simulink model "ASMC_withoutBP"  (R2020b)
settings: Solver=ode45  StartTime=0.0  StopTime=20  FixedStep=0.001  RelTol=1e-3
settings Model: Creator=cyx  LastModifiedBy=cyx
settings SolverCC: AlgebraicLoopSolver=LineSearch
settings DataIOCC: ReturnWorkspaceOutputs=off

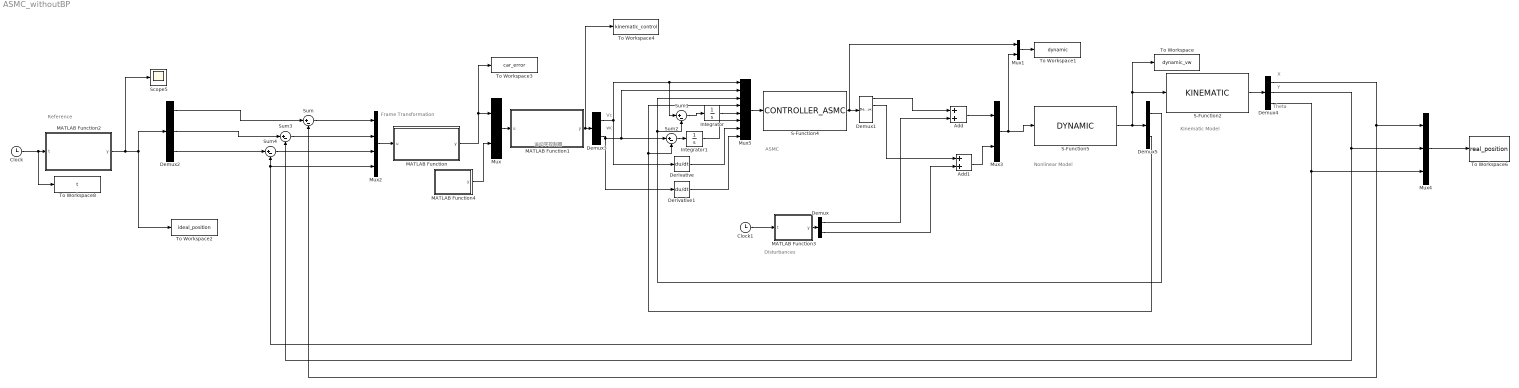
== system ASMC_withoutBP ==
  note: Y
  note: X
  note: Disturbances
  note: Reference
  note: Nonlinear Model
  note: ASMC
  note: 运动学控制器
  note: Kinematic Model
  note: Theta
  note: Vc
  note: Frame Transformation
  note: wc
  Add : Sum
  Add1 : Sum
  Clock : Clock
  Clock1 : Clock
  Demux : Demux  Outputs=2
  Demux1 : Demux
  Demux2 : Demux  Outputs=3
  Demux3 : Demux  Outputs=2
  Demux4 : Demux  Outputs=3
  Demux5 : Demux  Outputs=2
  Derivative : Derivative
  Derivative1 : Derivative
  Integrator : Integrator
  Integrator1 : Integrator
  MATLAB Function : MATLAB Function  TreatAsAtomicUnit=on
  MATLAB Function1 : MATLAB Function  TreatAsAtomicUnit=on
  MATLAB Function2 : MATLAB Function  TreatAsAtomicUnit=on
  MATLAB Function3 : MATLAB Function  TreatAsAtomicUnit=on
  MATLAB Function4 : MATLAB Function  TreatAsAtomicUnit=on
  Mux : Mux  Inputs=2
  Mux1 : Mux  Inputs=2
  Mux2 : Mux
  Mux3 : Mux  Inputs=2
  Mux4 : Mux  Inputs=3
  Mux5 : Mux  Inputs=8
  S-Function2 : S-Function  FunctionName=KINEMATIC  SFunctionDeploymentMode=off  EnableBusSupport=off
  S-Function4 : S-Function  FunctionName=CONTROLLER_ASMC  SFunctionDeploymentMode=off  EnableBusSupport=off
  S-Function5 : S-Function  FunctionName=DYNAMIC  SFunctionDeploymentMode=off  EnableBusSupport=off
  Scope5 : Scope
  Sum{,1..4} (5 alike) : Sum  Inputs=|+-
  To Workspace : ToWorkspace  VariableName=dynamic_vw  SampleTime=-1
  To Workspace1 : ToWorkspace  VariableName=dynamic  SampleTime=-1
  To Workspace2 : ToWorkspace  VariableName=ideal_position  SampleTime=-1
  To Workspace3 : ToWorkspace  VariableName=car_error  SampleTime=-1
  To Workspace4 : ToWorkspace  VariableName=kinematic_control  SampleTime=-1
  To Workspace6 : ToWorkspace  VariableName=real_position  SampleTime=-1
      settings: Save2DSignal=2-D array (concatenate along first dimension)
  To Workspace8 : ToWorkspace  VariableName=t  SampleTime=-1
  wires:
  Sum1/1 -> Integrator/1
  Demux3/1 -> Derivative/1, Sum1/1, Mux5/1
  Integrator1/1 -> Mux5/6
  Demux/2 -> Add1/2
  Integrator/1 -> Mux5/5
  Clock1/1 -> MATLAB Function3/1(t)
  Mux5/1 -> S-Function4/1
  Derivative1/1 -> Mux5/8
  Derivative/1 -> Mux5/7
  Sum2/1 -> Integrator1/1
  Demux3/2 -> Derivative1/1, Mux5/2, Sum2/1
  Demux1/1 -> Add/1
  Demux/1 -> Add/2
  S-Function5/1 -> S-Function2/1, To Workspace/1, Demux5/1
  Mux2/1 -> MATLAB Function/1(u)
  S-Function4/1 -> Mux1/1, Demux1/1
  Add1/1 -> Mux3/2
  Sum4/1 -> Mux2/3
  Sum3/1 -> Mux2/2
  MATLAB Function3/1(y) -> Demux/1
  Demux5/2 -> Mux5/4, Sum2/2
  Mux/1 -> MATLAB Function1/1(u)
  MATLAB Function/1(y) -> To Workspace3/1, Mux/1
  Demux1/2 -> Add1/1
  Clock/1 -> To Workspace8/1, MATLAB Function2/1(t)
  Demux5/1 -> Sum1/2, Mux5/3
  Mux4/1 -> To Workspace6/1
  Add/1 -> Mux3/1
  MATLAB Function2/1(y) -> Scope5/1, To Workspace2/1, Demux2/1
  Demux2/3 -> Sum4/1
  Demux2/2 -> Sum3/1
  Demux2/1 -> Sum/1
  Sum/1 -> Mux2/1
  MATLAB Function1/1(y) -> To Workspace4/1, Demux3/1
  Demux4/3 -> Mux2/4, Sum4/2, Mux4/3
  Demux4/1 -> Mux4/1, Sum/2
  S-Function2/1 -> Demux4/1
  Demux4/2 -> Sum3/2, Mux4/2
  MATLAB Function4/1(y) -> Mux/2
  Mux3/1 -> S-Function5/1, Mux1/2
  Mux1/1 -> To Workspace1/1

== matlab function ASMC_withoutBP/MATLAB Function ==
  data: u input; y output
function y = fcn(u)
%% ERROR TRANSFORMATION；
%转换矩阵C

C=[cos(u(4))   sin(u(4))      0;
    -sin(u(4)) cos(u(4))    0;
    0            0          1];

ex=C(1,1)*u(1)+C(1,2)*u(2);
ey=C(2,1)*u(1)+C(2,2)*u(2);
e_th=C(3,3)*u(3);
y =[ex;ey;e_th];

== matlab function ASMC_withoutBP/MATLAB Function2 ==
  data: t input; y output
function y = input(t)
x_r=t;
y_r=sin(t);
theta_r=0;

y =[x_r; y_r; theta_r];

== matlab function ASMC_withoutBP/MATLAB Function3 ==
  data: y output; t input
function y = fcn(t)

deta1=0.5*sin(3*t);
deta2=0.75*cos(2*t);

y =[deta1;deta2];

== matlab function ASMC_withoutBP/MATLAB Function4 ==
  data: y output
function y = fcn()

%% 经过BP优化的最终值
Kx=2;
Ky=150;
Ktheta=5;

y =[Kx;Ky;Ktheta];

== matlab function ASMC_withoutBP/MATLAB Function1 ==
  data: u input; y output
function y = kinematic_controller(u)

%% CONTROL INPUT
e_x=u(1);
e_y=u(2);
e_theta=u(3);
Kx=u(4);
Ky=u(5);
Ktheta=u(6);

v_r=0.06;w_r=0; %Desired linear and angular velocity 
%% --------Backstepping Kinematic Controller---------
v_c=v_r*cos(e_theta)+Kx*e_x;
w_c=w_r+Ky*v_r*e_y+Ktheta*v_r*sin(e_theta);

y = [v_c;w_c];
